simulink model "W6_cs"  (Simulink 8.3)
settings: Solver=ode4  SolverMode=SingleTasking  StartTime=0.0  StopTime=inf  FixedStep=1/60  RelTol=1e-3
PreLoadFcn:
  | check_NUTS_defined;
  | 
  | assignin('base',['model_closed_' bdroot],false);
InitFcn:
  | PreScanExperimentInitFcn(bdroot)
StopFcn:
  | PreScanExperimentStopFcn(bdroot)
  | close all;
  | 
  | format shortg
  | c = clock;
  | log_filename = ['log_EXT_',num2str(c(1)),'_',num2str(c(2)),'_',num2str(c(3)),'_',num2str(c(4)),'_',num2str(c(5)),'_',num2str(round(c(6)))];
  | save(log_filename,'res')
undefined symbols (not defined in the file): DiscIntNeverNeededParam, gray, warningInitialVelocity, x0
libraries: simulink x39, PreScanSimulinkLibrary x19, PreScanUsefulBlocks x10, simulink_extras x3, visionsources x2, dspsigops x2, dspnetwork x1, vrlib x1, visionsinks x1
(part 6 of 6)

== matlab function Audi_A8_1/Speedometer/MATLAB Function ==
  data: score input double
function Speedometer(score)
%#codegen

cla;
radius = 1; %unit circle
angle = -0.2*pi:0.05:1.2*pi; % for only a half circle
x = 0.025+radius * cos(angle);
y = -0.2+radius * sin(angle);
z = zeros(size(x));
col = x;  % This is the color, vary with x in this case.
surface([x;x],[y;y],[z;z],[col;col],'FaceColor','no','EdgeColor','none','LineWidth',45); %line width set to 45 since we need a thick line - can change this to anything
axis equal
axis off
hold on
scoreRange = linspace(1,0,length(angle));
[~,index] = min(abs(scoreRange - score));
plot([x(index),0],[y(index),0],'-','LineWidth',5,'Color','red')

end

== matlab function Audi_A8_1/PathFollower_Preview_1/LateralController/CTRL REFERENCES/Calculate Lateral Error/eml_find_10k_lateral_error_points ==
  data: pvp input double size=2; dist_psvehicle output double size=10; TrajOffset_x_y_Y input double size=3; ActorOffset_Left_Right input double; p0 input double size=2; PreviewDistance input double size=10; Traj_x parameter double; Traj_y parameter double; Traj_t parameter double; Traj_v parameter double; RefreshCounter parameter double
function dist_psvehicle  = eml_find_10k_lateral_error_points(pvp,TrajOffset_x_y_Y,ActorOffset_Left_Right,p0,PreviewDistance,Traj_x,Traj_y,Traj_t,Traj_v,RefreshCounter)

dist_psvehicle = emlfcn_find_10k_lateral_error_points(pvp,TrajOffset_x_y_Y,ActorOffset_Left_Right,p0,PreviewDistance,Traj_x,Traj_y,Traj_t,Traj_v,RefreshCounter);

% end function

== matlab function Audi_A8_1/Eye tracking/Driver Normal1 ==
  data: u input double; y output double
function y = fcn(u)
%#codegen
if u(7)> 0 && u(8)>0
    y = 0;
else
    y = 1;
end

== matlab function Audi_A8_1/PathFollower_Preview_1/LateralController/CTRL REFERENCES/Find Reference Point (pref0) on Trajectory closest to P0 Point (p0)/eml_find_closest_trajectory_points0 ==
  data: pvp input double size=2; Actor_traj_distance output double; TrajOffset_x_y_Y input double size=3; ActorOffset_Left_Right input double; p0 input double size=3; Traj_x parameter double; Traj_y parameter double; Actor_traj_angle output double; RefreshCounter parameter double
function [Actor_traj_distance,Actor_traj_angle]  = eml_find_closest_trajectory_points0(pvp,TrajOffset_x_y_Y,ActorOffset_Left_Right,p0,Traj_x,Traj_y,RefreshCounter)

[Actor_traj_distance,Actor_traj_angle]  = emlfcn_find_closest_trajectory_points0(pvp,TrajOffset_x_y_Y,ActorOffset_Left_Right,p0,Traj_x,Traj_y,RefreshCounter);

% end function

== matlab function Audi_A8_1/PathFollower_Preview_1/LateralController/Calculate delta steering error/eml_delta_steering_error ==
  data: v_x_vehicle input double; v_x_vehicle_Min input double; t_Preview_LatCtrl input double; delta_steeringwheeltotal output double; v_y_vehicle input double; yawrate_vehicle input double; CorneringStiffness_Tyres_Front input double; CorneringStiffness_Tyres_Rear input double; m_vehicle_total input double; inertia_z_vehicle_total input double; e_Lat input double size=10; Pos_x_CoG_Vehicle input double; wheelbase input double; RefreshCounter parameter double
function delta_steeringwheeltotal = eml_delta_steering_error(v_x_vehicle,v_x_vehicle_Min,t_Preview_LatCtrl,v_y_vehicle,yawrate_vehicle,CorneringStiffness_Tyres_Front,CorneringStiffness_Tyres_Rear,m_vehicle_total,inertia_z_vehicle_total,e_Lat,Pos_x_CoG_Vehicle,wheelbase,RefreshCounter)

delta_steeringwheeltotal = emlfcn_delta_steering_error(v_x_vehicle,v_x_vehicle_Min,t_Preview_LatCtrl,v_y_vehicle,yawrate_vehicle,CorneringStiffness_Tyres_Front,CorneringStiffness_Tyres_Rear,m_vehicle_total,inertia_z_vehicle_total,e_Lat,Pos_x_CoG_Vehicle,wheelbase,RefreshCounter);

% end function
